simulink model "S_GRAF_EXP_FL_EHGO_P_V1"  (R2017a)
settings: Solver=VariableStepAuto  StartTime=0.0  StopTime=inf  RelTol=1e-3
undefined symbols (not defined in the file or in its folder): serial
libraries: instrumentlib x3, simulink x1
settings Model: Creator=dricl  LastModifiedBy=dricl

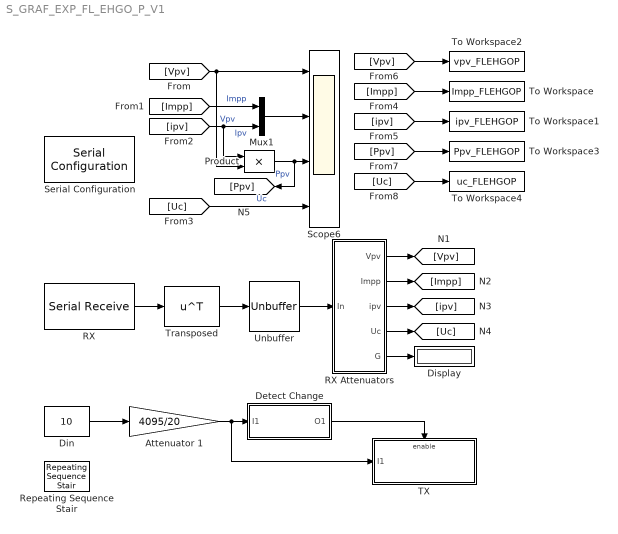
== system S_GRAF_EXP_FL_EHGO_P_V1 ==
  Attenuator 1 : Gain  Gain=4095/20  OutDataTypeStr=uint16
  Detect Change : Subsystem
  Din : Constant  Value=10  VectorParams1D=off  OutDataTypeStr=double  SampleTime=0.03
  Display : Display
  Mux1 : Mux  Inputs=2
  Product : Product
  RX : instrumentlib/Serial Receive  ComPortMenu=<Please select a port...>  ComPort=COM4  ObjConstructor=serial('COM4');  Header=SS  Terminator=EE  DataSize="[5  600]"  DataType=uint16  EnableBlockingMode=on  ActionDataUnavailable=Output custom value  CustomValue=3  SampleTime=0.03
  RX Attenuators : Subsystem
  Repeating Sequence Stair : simulink/Sources/Repeating Sequence Stair  OutValues=[0.6, 2, 0.8, 1.8].'  tsamp=1  OutMin=[]  OutMax=[]  OutDataTypeStr=double  OutputDataTypeScalingMode=double  OutDataType=fixdt(0,8)  ConRadixGroup=Best Precision: Vector-wise  OutScaling=2^-12
  Scope6 : Scope  NumInputPorts=4
  Serial Configuration : instrumentlib/Serial Configuration  Priority=-200000  ComPortMenu=<Please select a port...>  ComPort=COM4  ObjConstructor=serial('COM4');  BaudRate=921600  DataBits=8  Parity=none  StopBits=1  FlowControl=none  Timeout=60  ByteOrder=LittleEndian
  TX : Subsystem  TreatAsAtomicUnit=on
  To Workspace : ToWorkspace  VariableName=Impp_FLEHGOP  SaveFormat=Timeseries  SampleTime=-1
  To Workspace1 : ToWorkspace  VariableName=ipv_FLEHGOP  SaveFormat=Timeseries  SampleTime=-1
  To Workspace2 : ToWorkspace  VariableName=vpv_FLEHGOP  SaveFormat=Timeseries  SampleTime=-1
  To Workspace3 : ToWorkspace  VariableName=Ppv_FLEHGOP  SaveFormat=Timeseries  SampleTime=-1
  To Workspace4 : ToWorkspace  VariableName=uc_FLEHGOP  SaveFormat=Timeseries  SampleTime=-1
  Transposed : Math  Operator=transpose  SaturateOnIntegerOverflow=on
  Unbuffer : Unbuffer
  wires:
  Unbuffer/1 -> RX Attenuators/1(In)
  RX Attenuators/4(Uc) -> [Uc]
  RX Attenuators/2(Impp) -> [Impp]
  RX Attenuators/3(ipv) -> [ipv]
  RX Attenuators/1(Vpv) -> [Vpv]
  Transposed/1 -> Unbuffer/1
  RX/1 -> Transposed/1
  [Vpv] -> Scope6/1, Product/2  "Vpv"
  Detect Change/1(O1) -> TX/Enable
  Attenuator 1/1 -> TX/1(I1), Detect Change/1(I1)
  RX Attenuators/5(G) -> Display/1
  Mux1/1 -> Scope6/2
  [ipv] -> Product/1, Mux1/2  "Ipv"
  [Impp] -> Mux1/1  "Impp"
  Din/1 -> Attenuator 1/1
  [Uc] -> Scope6/4  "Uc"
  Product/1 -> [Ppv], Scope6/3  "Ppv"
  [Impp] -> To Workspace/1
  [ipv] -> To Workspace1/1
  [Vpv] -> To Workspace2/1
  [Ppv] -> To Workspace3/1
  [Uc] -> To Workspace4/1

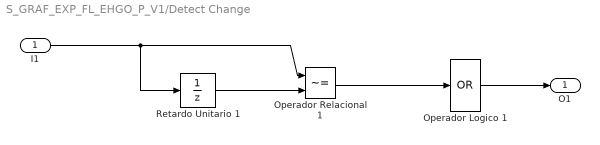
== system S_GRAF_EXP_FL_EHGO_P_V1/Detect Change ==
  I1 : Inport
  Operador Logico 1 : Logic  Operator=OR  Inputs=1  AllPortsSameDT=off  OutDataTypeStr=boolean
  Operador Relacional 1 : RelationalOperator  Operator=~=  OutDataTypeStr=boolean  RndMeth=Nearest
  Retardo Unitario 1 : UnitDelay  InitialCondition=0.5  SampleTime=0.1
  O1 : Outport
  wires:
  Retardo Unitario 1/1 -> Operador Relacional 1/2
  I1/1 -> Operador Relacional 1/1, Retardo Unitario 1/1
  Operador Relacional 1/1 -> Operador Logico 1/1
  Operador Logico 1/1 -> O1/1

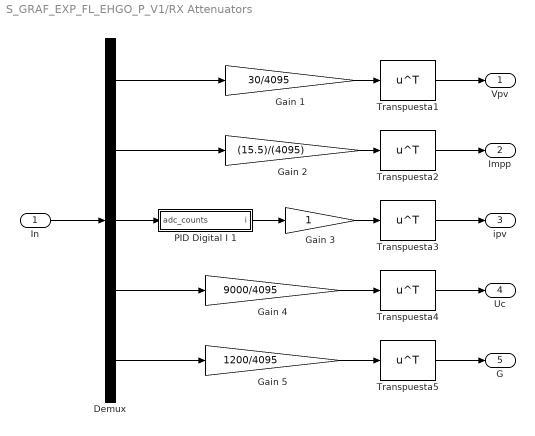
== system S_GRAF_EXP_FL_EHGO_P_V1/RX Attenuators ==
  In : Inport
  Demux : Demux  Outputs=5
  Gain 1 : Gain  Gain=30/4095  OutDataTypeStr=double
  Gain 2 : Gain  Gain=(15.5)/(4095)  OutDataTypeStr=double
  Gain 3 : Gain  OutDataTypeStr=double
  Gain 4 : Gain  Gain=9000/4095  OutDataTypeStr=double
  Gain 5 : Gain  Gain=1200/4095  OutDataTypeStr=double
  PID Digital I 1 : MATLAB Function  TreatAsAtomicUnit=on
  Transpuesta{1..5} (5 alike) : Math  Operator=transpose  SaturateOnIntegerOverflow=on
  Vpv : Outport
  Impp : Outport  Port=2
  ipv : Outport  Port=3
  Uc : Outport  Port=4
  G : Outport  Port=5
  wires:
  Transpuesta2/1 -> Impp/1
  Gain 1/1 -> Transpuesta1/1
  Demux/1 -> Gain 1/1
  In/1 -> Demux/1
  Transpuesta1/1 -> Vpv/1
  Gain 2/1 -> Transpuesta2/1
  Demux/2 -> Gain 2/1
  Gain 3/1 -> Transpuesta3/1
  Transpuesta3/1 -> ipv/1
  Demux/3 -> PID Digital I 1/1(adc_counts)
  Demux/4 -> Gain 4/1
  Gain 4/1 -> Transpuesta4/1
  Demux/5 -> Gain 5/1
  Gain 5/1 -> Transpuesta5/1
  PID Digital I 1/1(i) -> Gain 3/1
  Transpuesta4/1 -> Uc/1
  Transpuesta5/1 -> G/1

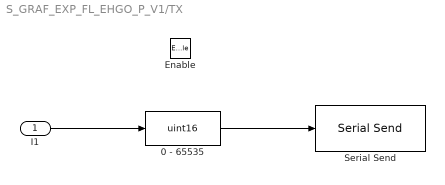
== system S_GRAF_EXP_FL_EHGO_P_V1/TX ==
  I1 : Inport
  Enable : EnablePort
  "0 - 65535 " : DataTypeConversion  OutDataTypeStr=uint16  ConvertRealWorld=Stored Integer (SI)
  Serial Send : instrumentlib/Serial Send  ComPortMenu=<Please select a port...>  ComPort=COM4  ObjConstructor=serial('COM4');  Terminator=<none>  EnableBlockingMode=off
  wires:
  I1/1 -> "0 - 65535 "/1
  "0 - 65535 "/1 -> Serial Send/1

== matlab function S_GRAF_EXP_FL_EHGO_P_V1/RX Attenuators/PID Digital I 1 ==
  data: adc_counts input; i output
function i = fcn(adc_counts)
% adc_counts: 0..4095
% i: corriente corregida (A)

ADCmax = 4095;

% Conversión ideal (datasheet)
i_raw = 36.7 * (double(adc_counts)/double(ADCmax)) - 18.3;

% Calibración con tus 2 puntos:
% i_raw(0A)=-0.5  y  i_raw(2A)=1.35
m = 2/1.85;                 % 1.081081081...
c = 0.5405405405405406;     % = m*0.5

i = m*i_raw + c;

% Saturación opcional
if i > 15.5
    i = 15.5;
elseif i < -15.5
    i = -15.5;
end

end
